simulink model "Tangentialkraftverteilung"  (R2023a)
settings: Solver=VariableStepAuto  StartTime=0.0  StopTime=10.0  RelTol=1e-3
model workspace (MAT data in the model file):
  h_s = 0.5
  l = 2.8
  l_v = 1.344
undefined symbols (not defined in the file or in its folder): hs, L, Lv
settings Model: Creator=lenan  LastModifiedBy=tinah
settings SolverCC: AlgebraicLoopSolver=TrustRegion
settings DebuggingCC: UnconnectedInputMsg=warning  UnconnectedOutputMsg=warning  UnconnectedLineMsg=warning
settings ModelReferenceCC: EnableRefExpFcnMdlSchedulingChecks=on

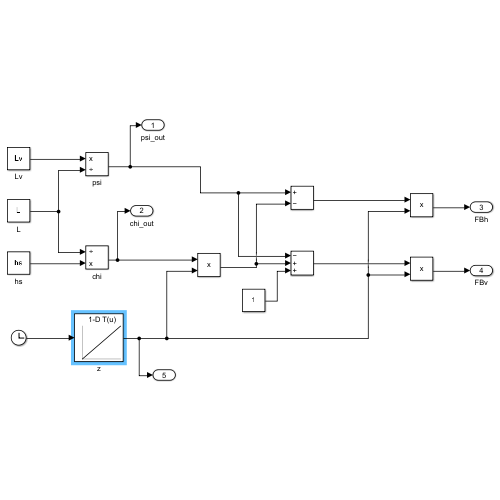
[thumbnail: Simulink's stored preview of the top-level diagram]
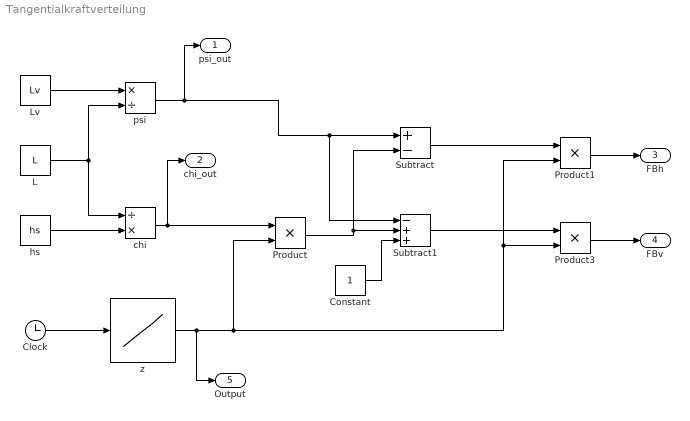
== system Tangentialkraftverteilung ==
  Clock : Clock
  Constant : Constant
  L : Constant  Value=L
  Lv : Constant  Value=Lv
  Product : Product
  Product1 : Product
  Product3 : Product
  Subtract : Sum  Inputs=+-
  Subtract1 : Sum  Inputs=-++
  chi : Product  Inputs=/*
  hs : Constant  Value=hs
  psi : Product  Inputs=*/
  z : Lookup_n-D  NumberOfTableDimensions=1  BreakpointsForDimension1=[0.01 ((Lv/l)/(hs/l))-(-(1-Lv/L)/(hs/L))]  Table=[(-(1-Lv/l)/(hs/L)) ((Lv/l)/(hs/L))]  InternalRulePriority=Speed  RndMeth=Simplest
  psi_out : Outport
  chi_out : Outport  Port=2
  FBh : Outport  Port=3
  FBv : Outport  Port=4
  Output : Outport  Port=5
  wires:
  Lv/1 -> psi/1
  L/1 -> chi/1, psi/2
  hs/1 -> chi/2
  Clock/1 -> z/1
  z/1 -> Output/1, Product/2, Product3/2, Product1/2
  chi/1 -> chi_out/1, Product/1
  psi/1 -> psi_out/1, Subtract1/1, Subtract/1
  Subtract/1 -> Product1/1
  Product/1 -> Subtract1/2, Subtract/2
  Constant/1 -> Subtract1/3
  Subtract1/1 -> Product3/1
  Product1/1 -> FBh/1
  Product3/1 -> FBv/1
